simulink library "lib_GRM_HIL"  (R2019b)
settings: Solver=VariableStepAuto  StartTime=0.0  StopTime=10.0  RelTol=1e-3
values from neighbouring files (symbols this model uses):
  HIL_Sample_Time = 0.001    [initialize_GRM_HIL.m]
undefined symbols (not defined in the file or in its folder): HIL_Data
libraries: simulink x4, lib_Servo x3, lib_Flight_Controller x3, lib_Gimbal x3, lib_Encoder x2, lib_Serial_PIX x2, lib_Gimbal_Ctrl x2, lib_FDM x2, lib_Fin_Deflections x1, lib_Gimbal_Cmd x1, lib_IMU_GPS_Emulator x1, sldrtlib x1
settings Model: Creator=m.hiepp  LastModifiedBy=guy-m
settings DataIOCC: ReturnWorkspaceOutputs=off
settings DebuggingCC: ArithmeticOperatorsInVariantConditions=warning
settings SFSimCC: CustomCodeUndefinedFunction=UseInterfaceOnly

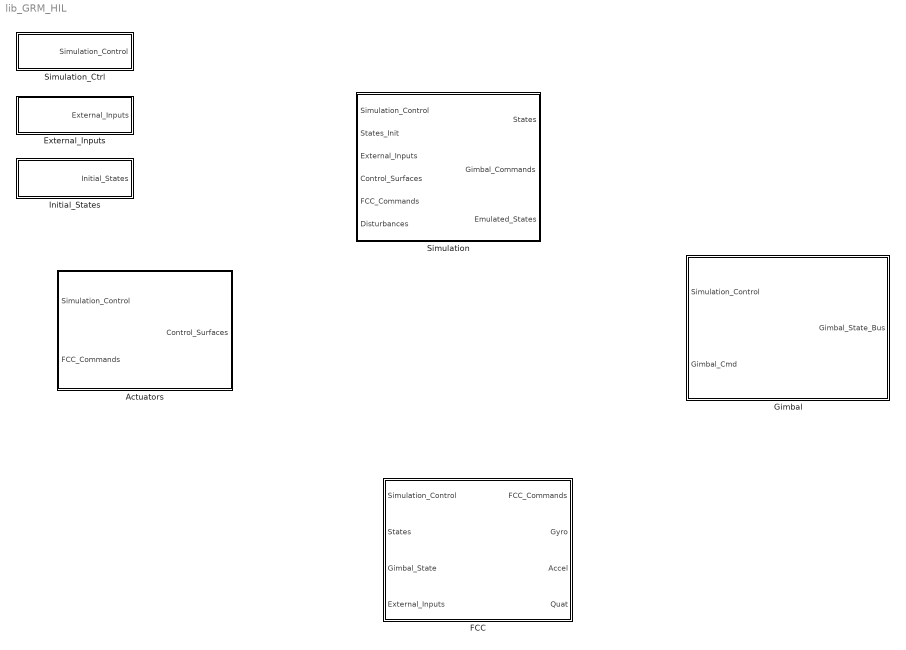
== system lib_GRM_HIL ==
  Actuators : Subsystem  Variant=on
  External_Inputs : Subsystem  mask{External_Inputs=HIL_Data.External_Inputs}
      mask prompts: External_Inputs "External Inputs Data"
  FCC : Subsystem  Variant=on
  Gimbal : Subsystem  Variant=on
  Initial_States : Subsystem  mask{Rigid_Body=HIL_Data.Initial_States.Rigid_Body, Airframe=HIL_Data.Initial_States.Airframe, Atm=HIL_Data.Initial_States.Atm}
      mask prompts: Rigid_Body "Rigid_Body Initial States Data"; Airframe "Airframe Initial States Data"; Atm "Atm Initial States Data"
  Simulation : Subsystem
  Simulation_Ctrl : Subsystem

== system lib_GRM_HIL/Actuators ==
  Simulation_Control : Inport  OutDataTypeStr=Bus: Simulation_Ctrl_Bus
  FCC_Commands : Inport  Port=2  OutDataTypeStr=Bus: FCC_Commands_Bus
  Emulate_Actuators : Subsystem  VariantControl=VSS_ACT_EMUL
  Use_Actuators : Subsystem  VariantControl=VSS_ACT_REAL
  Control_Surfaces : Outport  OutDataTypeStr=Bus: Control_Surface_Bus  VectorParamsAs1DForOutWhenUnconnected=off

== system lib_GRM_HIL/External_Inputs ==
  note: actually commanding roll rate instead of bank angle!!
  Bus Creator : BusCreator  Inputs=2  OutDataTypeStr=Bus: External_Inputs_Bus
  Bus Creator1 : BusCreator  Inputs=1  OutDataTypeStr=Bus: FDM_External_Inputs_Bus
  Bus Creator2 : BusCreator  Inputs=4  OutDataTypeStr=Bus: FCC_External_Inputs_Bus
  Commands_Generator : Subsystem
  Constant1 : Constant  Value=External_Inputs.FCC.Flight_Termination_flg  OutDataTypeStr=boolean
  Data Type Conversion : DataTypeConversion  OutDataTypeStr=boolean
  Step : Step  Time=External_Inputs.FDM.Motor_Ignition_time_s  SampleTime=0
  External_Inputs : Outport  OutDataTypeStr=Bus: External_Inputs_Bus  VectorParamsAs1DForOutWhenUnconnected=off
  wires:
  Bus Creator/1 -> External_Inputs/1
  Bus Creator1/1 -> Bus Creator/1  "FDM_External_Inputs_Bus"
  Bus Creator2/1 -> Bus Creator/2  "FCC_External_Inputs_Bus"
  Constant1/1 -> Bus Creator2/1  "Flight_Termination_flg"
  Step/1 -> Data Type Conversion/1
  Data Type Conversion/1 -> Bus Creator1/1  "Motor_Ignition_flg"
  Commands_Generator/3(CMD_acc_y_mDs2) -> Bus Creator2/4  "CMD_acc_y_mDs2"
  Commands_Generator/2(CMD_acc_z_mDs2) -> Bus Creator2/3  "CMD_acc_z_mDs2"
  Commands_Generator/1(CMD_phi_rad) -> Bus Creator2/2  "CMD_phi_rad"

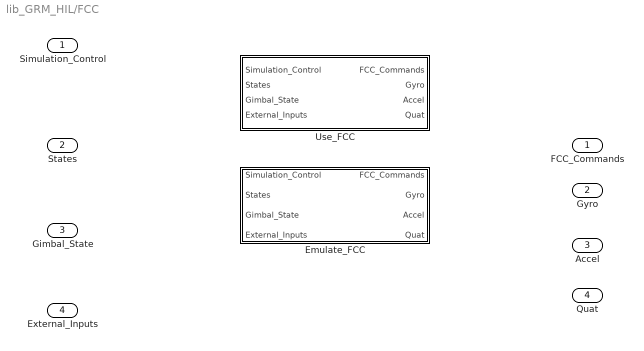
== system lib_GRM_HIL/FCC ==
  Simulation_Control : Inport  OutDataTypeStr=Bus: Simulation_Ctrl_Bus
  States : Inport  Port=2  OutDataTypeStr=Bus: States_Bus
  Gimbal_State : Inport  Port=3  OutDataTypeStr=Bus: Gimbal_State_Bus
  External_Inputs : Inport  Port=4  OutDataTypeStr=Bus: External_Inputs_Bus
  Emulate_FCC : Subsystem  VariantControl=VSS_FCC_EMUL
  Use_FCC : Subsystem  VariantControl=VSS_FCC_REAL
  FCC_Commands : Outport  OutDataTypeStr=Bus: FCC_Commands_Bus  VectorParamsAs1DForOutWhenUnconnected=off
  Gyro : Outport  Port=2
  Accel : Outport  Port=3
  Quat : Outport  Port=4

== system lib_GRM_HIL/Gimbal ==
  Simulation_Control : Inport  OutDataTypeStr=Bus: Simulation_Ctrl_Bus
  Gimbal_Cmd : Inport  Port=2  OutDataTypeStr=Bus: Gimbal_Cmd_Bus
  Emulate_Gimbal : Subsystem  VariantControl=VSS_GIMBAL_EMUL
  Use_Gimbal : Subsystem  VariantControl=VSS_GIMBAL_REAL
  Use_Gimbal_HWInterface_CC : Subsystem  VariantControl=VSS_GIMBAL_HWICC
  Gimbal_State_Bus : Outport  OutDataTypeStr=Bus: Gimbal_State_Bus  VectorParamsAs1DForOutWhenUnconnected=off

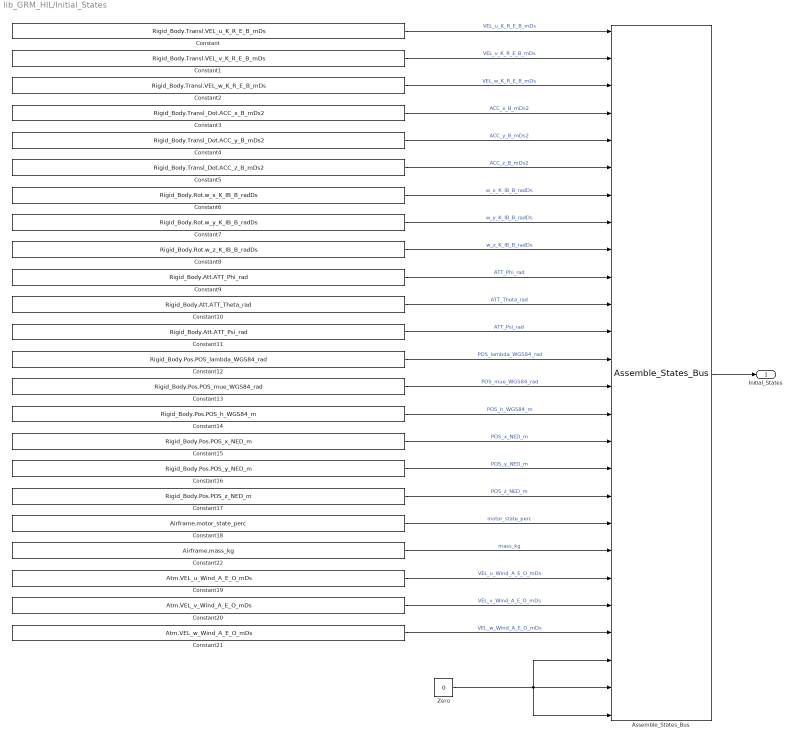
== system lib_GRM_HIL/Initial_States ==
  Assemble_States_Bus : lib_FDM/Assemble_States_Bus  SystemSampleTime=-1  Latency=0  AutoFrameSizeCalculation=off
  Constant : Constant  Value=Rigid_Body.Transl.VEL_u_K_R_E_B_mDs
  Constant1 : Constant  Value=Rigid_Body.Transl.VEL_v_K_R_E_B_mDs
  Constant10 : Constant  Value=Rigid_Body.Att.ATT_Theta_rad
  Constant11 : Constant  Value=Rigid_Body.Att.ATT_Psi_rad
  Constant12 : Constant  Value=Rigid_Body.Pos.POS_lambda_WGS84_rad
  Constant13 : Constant  Value=Rigid_Body.Pos.POS_mue_WGS84_rad
  Constant14 : Constant  Value=Rigid_Body.Pos.POS_h_WGS84_m
  Constant15 : Constant  Value=Rigid_Body.Pos.POS_x_NED_m
  Constant16 : Constant  Value=Rigid_Body.Pos.POS_y_NED_m
  Constant17 : Constant  Value=Rigid_Body.Pos.POS_z_NED_m
  Constant18 : Constant  Value=Airframe.motor_state_perc
  Constant19 : Constant  Value=Atm.VEL_u_Wind_A_E_O_mDs
  Constant2 : Constant  Value=Rigid_Body.Transl.VEL_w_K_R_E_B_mDs
  Constant20 : Constant  Value=Atm.VEL_v_Wind_A_E_O_mDs
  Constant21 : Constant  Value=Atm.VEL_w_Wind_A_E_O_mDs
  Constant22 : Constant  Value=Airframe.mass_kg
  Constant3 : Constant  Value=Rigid_Body.Transl_Dot.ACC_x_B_mDs2
  Constant4 : Constant  Value=Rigid_Body.Transl_Dot.ACC_y_B_mDs2
  Constant5 : Constant  Value=Rigid_Body.Transl_Dot.ACC_z_B_mDs2
  Constant6 : Constant  Value=Rigid_Body.Rot.w_x_K_IB_B_radDs
  Constant7 : Constant  Value=Rigid_Body.Rot.w_y_K_IB_B_radDs
  Constant8 : Constant  Value=Rigid_Body.Rot.w_z_K_IB_B_radDs
  Constant9 : Constant  Value=Rigid_Body.Att.ATT_Phi_rad
  Zero : Constant  Value=0  OutDataTypeStr=Inherit: Inherit via back propagation
  Initial_States : Outport  OutDataTypeStr=Bus: States_Bus  VectorParamsAs1DForOutWhenUnconnected=off
  wires:
  Assemble_States_Bus/1 -> Initial_States/1
  Constant/1 -> Assemble_States_Bus/1  "VEL_u_K_R_E_B_mDs"
  Constant1/1 -> Assemble_States_Bus/2  "VEL_v_K_R_E_B_mDs"
  Constant2/1 -> Assemble_States_Bus/3  "VEL_w_K_R_E_B_mDs"
  Constant4/1 -> Assemble_States_Bus/5  "ACC_y_B_mDs2"
  Constant3/1 -> Assemble_States_Bus/4  "ACC_x_B_mDs2"
  Constant5/1 -> Assemble_States_Bus/6  "ACC_z_B_mDs2"
  Constant6/1 -> Assemble_States_Bus/7  "w_x_K_IB_B_radDs"
  Constant7/1 -> Assemble_States_Bus/8  "w_y_K_IB_B_radDs"
  Constant8/1 -> Assemble_States_Bus/9  "w_z_K_IB_B_radDs"
  Constant9/1 -> Assemble_States_Bus/10  "ATT_Phi_rad"
  Constant10/1 -> Assemble_States_Bus/11  "ATT_Theta_rad"
  Constant11/1 -> Assemble_States_Bus/12  "ATT_Psi_rad"
  Constant12/1 -> Assemble_States_Bus/13  "POS_lambda_WGS84_rad"
  Constant13/1 -> Assemble_States_Bus/14  "POS_mue_WGS84_rad"
  Constant14/1 -> Assemble_States_Bus/15  "POS_h_WGS84_m"
  Constant15/1 -> Assemble_States_Bus/16  "POS_x_NED_m"
  Constant16/1 -> Assemble_States_Bus/17  "POS_y_NED_m"
  Constant17/1 -> Assemble_States_Bus/18  "POS_z_NED_m"
  Constant18/1 -> Assemble_States_Bus/19  "motor_state_perc"
  Constant19/1 -> Assemble_States_Bus/21  "VEL_u_Wind_A_E_O_mDs"
  Constant21/1 -> Assemble_States_Bus/23  "VEL_w_Wind_A_E_O_mDs"
  Constant20/1 -> Assemble_States_Bus/22  "VEL_v_Wind_A_E_O_mDs"
  Constant22/1 -> Assemble_States_Bus/20  "mass_kg"
  Zero/1 -> Assemble_States_Bus/26, Assemble_States_Bus/25, Assemble_States_Bus/24

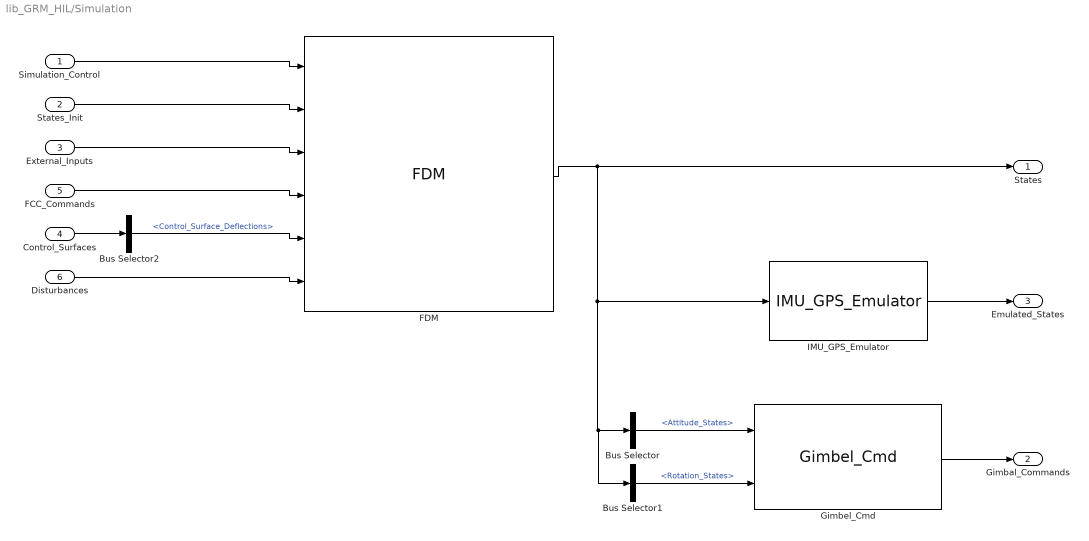
== system lib_GRM_HIL/Simulation ==
  Simulation_Control : Inport  OutDataTypeStr=Bus: Simulation_Ctrl_Bus
  States_Init : Inport  Port=2  OutDataTypeStr=Bus: States_Bus
  External_Inputs : Inport  Port=3  OutDataTypeStr=Bus: External_Inputs_Bus
  Control_Surfaces : Inport  Port=4  OutDataTypeStr=Bus: Control_Surface_Bus
  FCC_Commands : Inport  Port=5  OutDataTypeStr=Bus: FCC_Commands_Bus
  Disturbances : Inport  Port=6  OutDataTypeStr=Bus: Disturbances_Bus
  Bus Selector : BusSelector  OutputSignals=Rigid_Body_States.Attitude_States
  Bus Selector1 : BusSelector  OutputSignals=Rigid_Body_States.Rotation_States
  Bus Selector2 : BusSelector  OutputSignals=Control_Surface_Deflections
  FDM : lib_FDM/FDM  SystemSampleTime=-1  Latency=0  AutoFrameSizeCalculation=off
  Gimbel_Cmd : lib_Gimbal_Cmd/Gimbel_Cmd  SystemSampleTime=-1  Latency=0  AutoFrameSizeCalculation=off
  IMU_GPS_Emulator : lib_IMU_GPS_Emulator/IMU_GPS_Emulator  SystemSampleTime=-1  Latency=0  AutoFrameSizeCalculation=off
  States : Outport  OutDataTypeStr=Bus: States_Bus  VectorParamsAs1DForOutWhenUnconnected=off
  Gimbal_Commands : Outport  Port=2  OutDataTypeStr=Bus: Gimbal_Cmd_Bus  VectorParamsAs1DForOutWhenUnconnected=off
  Emulated_States : Outport  Port=3  OutDataTypeStr=Bus: States_Bus  VectorParamsAs1DForOutWhenUnconnected=off
  wires:
  FDM/1 -> Bus Selector/1, Bus Selector1/1, IMU_GPS_Emulator/1, States/1
  IMU_GPS_Emulator/1 -> Emulated_States/1
  Gimbel_Cmd/1 -> Gimbal_Commands/1
  Bus Selector/1 -> Gimbel_Cmd/1  "<Attitude_States>"
  Bus Selector1/1 -> Gimbel_Cmd/2  "<Rotation_States>"
  Simulation_Control/1 -> FDM/1
  States_Init/1 -> FDM/2
  External_Inputs/1 -> FDM/3
  FCC_Commands/1 -> FDM/4
  Control_Surfaces/1 -> Bus Selector2/1
  Bus Selector2/1 -> FDM/5  "<Control_Surface_Deflections>"
  Disturbances/1 -> FDM/6

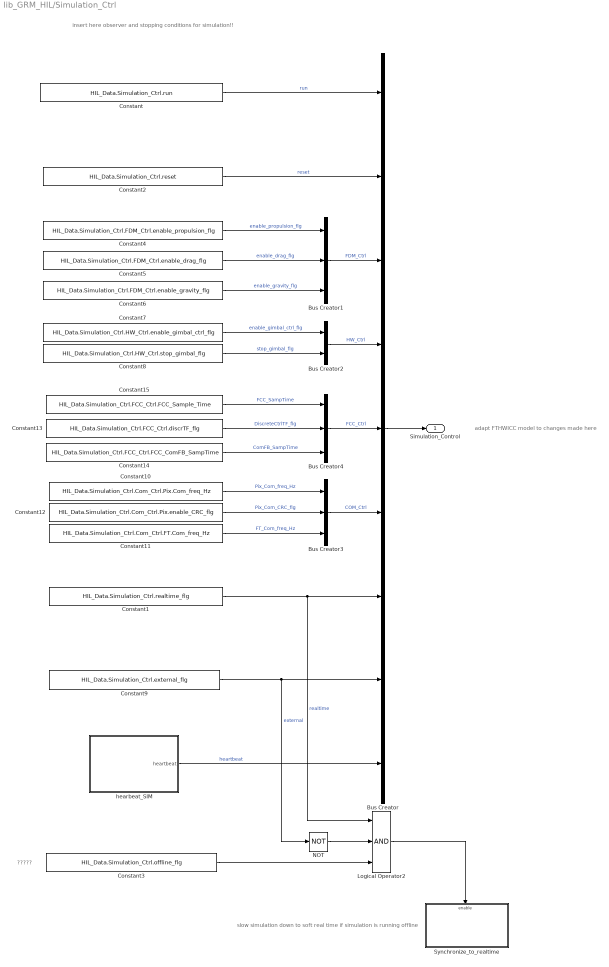
== system lib_GRM_HIL/Simulation_Ctrl ==
  note: adapt FTHWICC model to changes made here
  note: ?????
  note: slow simulation down to soft real time if simulation is running offline
  note: insert here observer and stopping conditions for simulation!!
  Bus Creator : BusCreator  Inputs=9  OutDataTypeStr=Bus: Simulation_Ctrl_Bus
  Bus Creator1 : BusCreator  Inputs=3  OutDataTypeStr=Bus: FDM_Ctrl_Bus
  Bus Creator2 : BusCreator  Inputs=2  OutDataTypeStr=Bus: HW_Ctrl_Bus
  Bus Creator3 : BusCreator  Inputs=3  OutDataTypeStr=Bus: COM_Ctrl_Bus
  Bus Creator4 : BusCreator  Inputs=3  OutDataTypeStr=Bus: FCC_Ctrl_Bus
  Constant : Constant  Value=HIL_Data.Simulation_Ctrl.run  OutDataTypeStr=boolean
  Constant1 : Constant  Value=HIL_Data.Simulation_Ctrl.realtime_flg  OutDataTypeStr=boolean
  Constant10 : Constant  Value=HIL_Data.Simulation_Ctrl.Com_Ctrl.Pix.Com_freq_Hz  OutDataTypeStr=double
  Constant11 : Constant  Value=HIL_Data.Simulation_Ctrl.Com_Ctrl.FT.Com_freq_Hz  OutDataTypeStr=double
  Constant12 : Constant  Value=HIL_Data.Simulation_Ctrl.Com_Ctrl.Pix.enable_CRC_flg  OutDataTypeStr=boolean
  Constant13 : Constant  Value=HIL_Data.Simulation_Ctrl.FCC_Ctrl.discrTF_flg  OutDataTypeStr=boolean
  Constant14 : Constant  Value=HIL_Data.Simulation_Ctrl.FCC_Ctrl.FCC_ComFB_SampTime  OutDataTypeStr=double
  Constant15 : Constant  Value=HIL_Data.Simulation_Ctrl.FCC_Ctrl.FCC_Sample_Time  OutDataTypeStr=double
  Constant2 : Constant  Value=HIL_Data.Simulation_Ctrl.reset  OutDataTypeStr=boolean
  Constant3 : Constant  Value=HIL_Data.Simulation_Ctrl.offline_flg  OutDataTypeStr=boolean
  Constant4 : Constant  Value=HIL_Data.Simulation_Ctrl.FDM_Ctrl.enable_propulsion_flg  OutDataTypeStr=boolean
  Constant5 : Constant  Value=HIL_Data.Simulation_Ctrl.FDM_Ctrl.enable_drag_flg  OutDataTypeStr=boolean
  Constant6 : Constant  Value=HIL_Data.Simulation_Ctrl.FDM_Ctrl.enable_gravity_flg  OutDataTypeStr=boolean
  Constant7 : Constant  Value=HIL_Data.Simulation_Ctrl.HW_Ctrl.enable_gimbal_ctrl_flg  OutDataTypeStr=double
  Constant8 : Constant  Value=HIL_Data.Simulation_Ctrl.HW_Ctrl.stop_gimbal_flg  OutDataTypeStr=double
  Constant9 : Constant  Value=HIL_Data.Simulation_Ctrl.external_flg  OutDataTypeStr=boolean
  Logical Operator2 : Logic  Inputs=3  AllPortsSameDT=off  OutDataTypeStr=boolean
  NOT : Logic  Operator=NOT  IconShape=distinctive  AllPortsSameDT=off  OutDataTypeStr=boolean
  Synchronize_to_realtime : Subsystem
  hearbeat_SIM : Subsystem  mask{heartbeat=HIL_Data.Simulation_Ctrl.heartbeat}
      mask prompts: heartbeat "Simulation heartbeat data"
  Simulation_Control : Outport  OutDataTypeStr=Bus: Simulation_Ctrl_Bus  VectorParamsAs1DForOutWhenUnconnected=off
  wires:
  Bus Creator/1 -> Simulation_Control/1
  Constant/1 -> Bus Creator/1  "run"
  Constant1/1 -> Logical Operator2/1, Bus Creator/7  "realtime"
  Constant2/1 -> Bus Creator/2  "reset"
  Constant3/1 -> Logical Operator2/3
  Logical Operator2/1 -> Synchronize_to_realtime/Enable
  Bus Creator1/1 -> Bus Creator/3  "FDM_Ctrl"
  Constant4/1 -> Bus Creator1/1  "enable_propulsion_flg"
  Constant5/1 -> Bus Creator1/2  "enable_drag_flg"
  Constant6/1 -> Bus Creator1/3  "enable_gravity_flg"
  Bus Creator2/1 -> Bus Creator/4  "HW_Ctrl"
  Constant8/1 -> Bus Creator2/2  "stop_gimbal_flg"
  Constant7/1 -> Bus Creator2/1  "enable_gimbal_ctrl_flg"
  Constant9/1 -> NOT/1, Bus Creator/8  "external"
  NOT/1 -> Logical Operator2/2
  Bus Creator3/1 -> Bus Creator/6  "COM_Ctrl"
  Constant11/1 -> Bus Creator3/3  "FT_Com_freq_Hz"
  Constant10/1 -> Bus Creator3/1  "Pix_Com_freq_Hz"
  hearbeat_SIM/1(heartbeat) -> Bus Creator/9  "heartbeat"
  Constant12/1 -> Bus Creator3/2  "Pix_Com_CRC_flg"
  Bus Creator4/1 -> Bus Creator/5  "FCC_Ctrl"
  Constant15/1 -> Bus Creator4/1  "FCC_SampTime"
  Constant13/1 -> Bus Creator4/2  "DiscreteCtrlTF_flg"
  Constant14/1 -> Bus Creator4/3  "ComFB_SampTime"

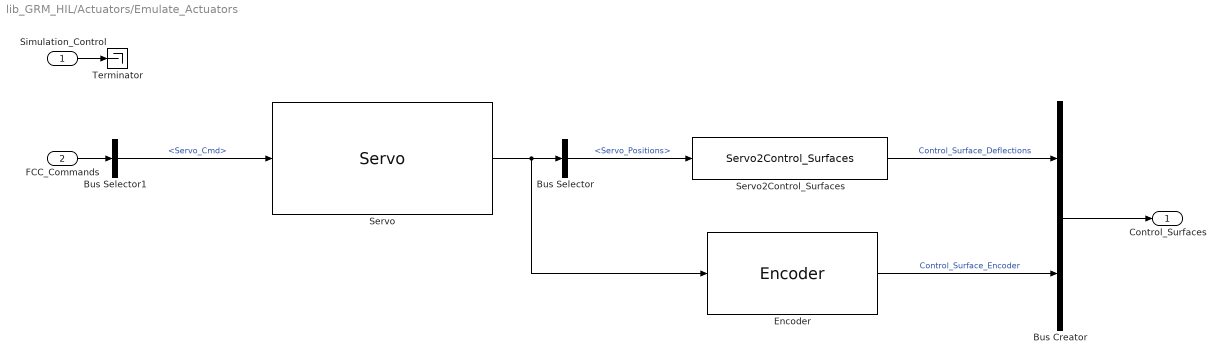
== system lib_GRM_HIL/Actuators/Emulate_Actuators ==
  Simulation_Control : Inport  OutDataTypeStr=Bus: Simulation_Ctrl_Bus
  FCC_Commands : Inport  Port=2  OutDataTypeStr=Bus: FCC_Commands_Bus
  Bus Creator : BusCreator  Inputs=2  OutDataTypeStr=Bus: Control_Surface_Bus
  Bus Selector : BusSelector  OutputSignals=Servo_Positions
  Bus Selector1 : BusSelector  OutputSignals=Airframe_Cmd.Servo_Cmd
  Encoder : lib_Encoder/Encoder  SystemSampleTime=-1  Latency=0  AutoFrameSizeCalculation=off
  Servo : lib_Servo/Servo  TF=HIL_Data.Servo.TF  PWM=HIL_Data.Servo.PWM
  Servo2Control_Surfaces : lib_Servo/Servo2Control_Surfaces  SystemSampleTime=-1  Latency=0  AutoFrameSizeCalculation=off
  Terminator : Terminator
  Control_Surfaces : Outport  OutDataTypeStr=Bus: Control_Surface_Bus  VectorParamsAs1DForOutWhenUnconnected=off
  wires:
  Encoder/1 -> Bus Creator/2  "Control_Surface_Encoder"
  Bus Creator/1 -> Control_Surfaces/1
  Bus Selector1/1 -> Servo/1  "<Servo_Cmd>"
  Servo2Control_Surfaces/1 -> Bus Creator/1  "Control_Surface_Deflections"
  Servo/1 -> Encoder/1, Bus Selector/1
  FCC_Commands/1 -> Bus Selector1/1
  Bus Selector/1 -> Servo2Control_Surfaces/1  "<Servo_Positions>"
  Simulation_Control/1 -> Terminator/1

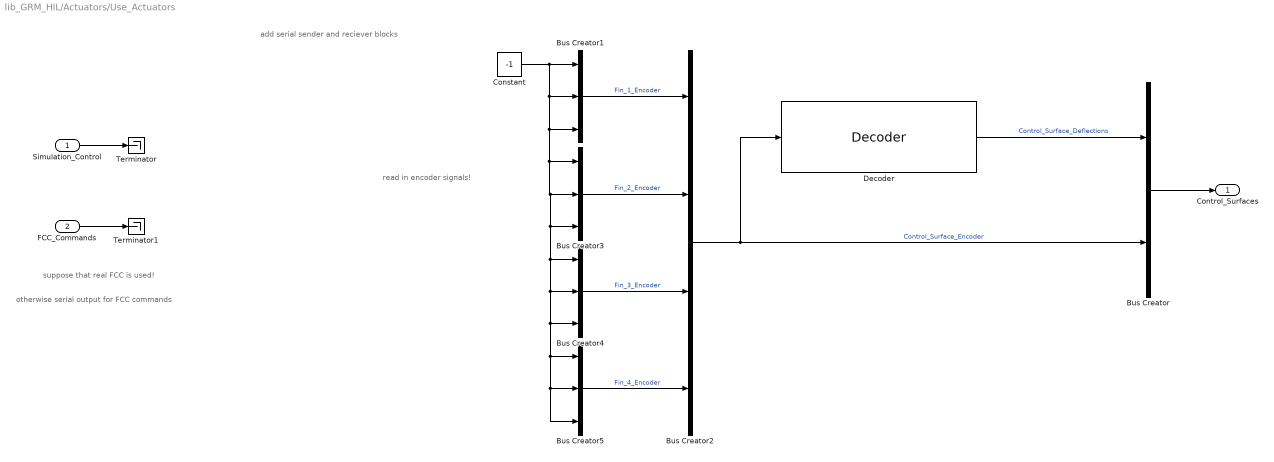
== system lib_GRM_HIL/Actuators/Use_Actuators ==
  note: read in encoder signals!
  note: otherwise serial output for FCC commands
  note: suppose that real FCC is used!
  note: add serial sender and reciever blocks
  Simulation_Control : Inport  OutDataTypeStr=Bus: Simulation_Ctrl_Bus
  FCC_Commands : Inport  Port=2  OutDataTypeStr=Bus: FCC_Commands_Bus
  Bus Creator : BusCreator  Inputs=2  OutDataTypeStr=Bus: Control_Surface_Bus
  Bus Creator{1,3..5} (4 alike) : BusCreator  Inputs=3  OutDataTypeStr=Bus: Inc_Encoder_Signal_Bus
  Bus Creator2 : BusCreator  Inputs=4  OutDataTypeStr=Bus: Control_Surface_Encoder_Bus
  Constant : Constant  Value=-1
  Decoder : lib_Encoder/Decoder  SystemSampleTime=-1  Latency=0  AutoFrameSizeCalculation=off
  Terminator : Terminator
  Terminator1 : Terminator
  Control_Surfaces : Outport  OutDataTypeStr=Bus: Control_Surface_Bus  VectorParamsAs1DForOutWhenUnconnected=off
  wires:
  Simulation_Control/1 -> Terminator/1
  FCC_Commands/1 -> Terminator1/1
  Bus Creator/1 -> Control_Surfaces/1
  Bus Creator2/1 -> Decoder/1, Bus Creator/2  "Control_Surface_Encoder"
  Bus Creator1/1 -> Bus Creator2/1  "Fin_1_Encoder"
  Bus Creator3/1 -> Bus Creator2/2  "Fin_2_Encoder"
  Bus Creator5/1 -> Bus Creator2/4  "Fin_4_Encoder"
  Bus Creator4/1 -> Bus Creator2/3  "Fin_3_Encoder"
  Decoder/1 -> Bus Creator/1  "Control_Surface_Deflections"
  Constant/1 -> Bus Creator4/1, Bus Creator5/1, Bus Creator5/3, Bus Creator5/2, Bus Creator4/3, Bus Creator4/2, Bus Creator3/3, Bus Creator3/2, Bus Creator3/1, Bus Creator1/3, Bus Creator1/2, Bus Creator1/1

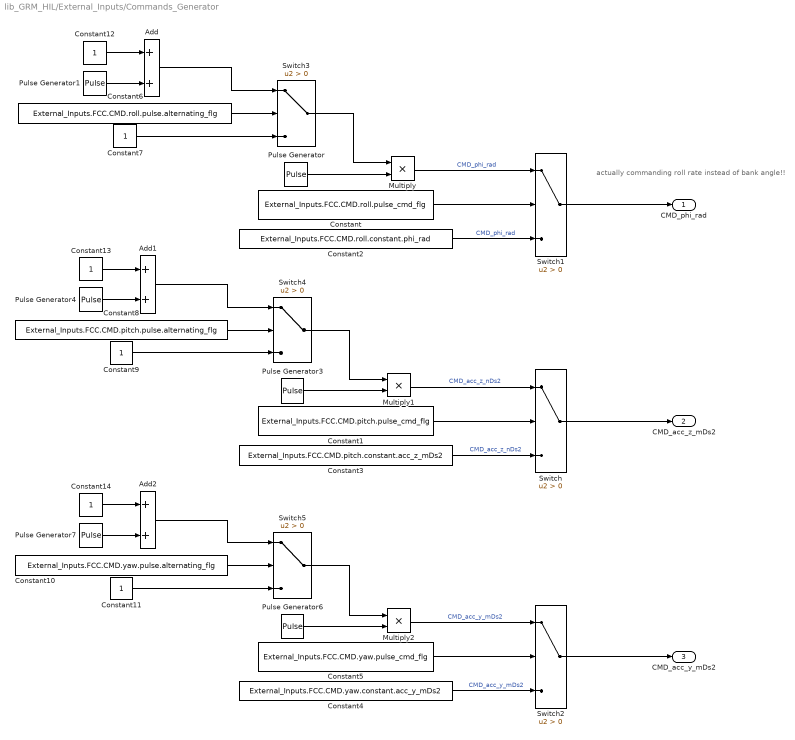
== system lib_GRM_HIL/External_Inputs/Commands_Generator ==
  note: actually commanding roll rate instead of bank angle!!
  Add : Sum
  Add1 : Sum
  Add2 : Sum
  Constant : Constant  Value=External_Inputs.FCC.CMD.roll.pulse_cmd_flg
  Constant1 : Constant  Value=External_Inputs.FCC.CMD.pitch.pulse_cmd_flg
  Constant10 : Constant  Value=External_Inputs.FCC.CMD.yaw.pulse.alternating_flg  OutDataTypeStr=boolean
  Constant{7,9,11..14} (6 alike) : Constant
  Constant2 : Constant  Value=External_Inputs.FCC.CMD.roll.constant.phi_rad
  Constant3 : Constant  Value=External_Inputs.FCC.CMD.pitch.constant.acc_z_mDs2
  Constant4 : Constant  Value=External_Inputs.FCC.CMD.yaw.constant.acc_y_mDs2
  Constant5 : Constant  Value=External_Inputs.FCC.CMD.yaw.pulse_cmd_flg
  Constant6 : Constant  Value=External_Inputs.FCC.CMD.roll.pulse.alternating_flg  OutDataTypeStr=boolean
  Constant8 : Constant  Value=External_Inputs.FCC.CMD.pitch.pulse.alternating_flg  OutDataTypeStr=boolean
  Multiply : Product
  Multiply1 : Product
  Multiply2 : Product
  Pulse Generator : DiscretePulseGenerator  PulseType=Time based  Amplitude=External_Inputs.FCC.CMD.roll.pulse.ampl_rad  Period=External_Inputs.FCC.CMD.roll.pulse.period_s  PulseWidth=External_Inputs.FCC.CMD.roll.pulse.pulse_width_perc  PhaseDelay=External_Inputs.FCC.CMD.roll.pulse.delay_s
  Pulse Generator1 : DiscretePulseGenerator  PulseType=Time based  Amplitude=-2  Period=2*External_Inputs.FCC.CMD.roll.pulse.period_s  PulseWidth=External_Inputs.FCC.CMD.roll.pulse.pulse_width_perc  PhaseDelay=External_Inputs.FCC.CMD.roll.pulse.delay_s+External_Inputs.FCC.CMD.roll.pulse.period_s
  Pulse Generator3 : DiscretePulseGenerator  PulseType=Time based  Amplitude=External_Inputs.FCC.CMD.pitch.pulse.ampl_mDs2  Period=External_Inputs.FCC.CMD.pitch.pulse.period_s  PulseWidth=External_Inputs.FCC.CMD.pitch.pulse.pulse_width_perc  PhaseDelay=External_Inputs.FCC.CMD.pitch.pulse.delay_s
  Pulse Generator4 : DiscretePulseGenerator  PulseType=Time based  Amplitude=-2  Period=2*External_Inputs.FCC.CMD.pitch.pulse.period_s  PulseWidth=External_Inputs.FCC.CMD.pitch.pulse.pulse_width_perc  PhaseDelay=External_Inputs.FCC.CMD.pitch.pulse.delay_s+External_Inputs.FCC.CMD.pitch.pulse.period_s
  Pulse Generator6 : DiscretePulseGenerator  PulseType=Time based  Amplitude=External_Inputs.FCC.CMD.yaw.pulse.ampl_mDs2  Period=External_Inputs.FCC.CMD.yaw.pulse.period_s  PulseWidth=External_Inputs.FCC.CMD.yaw.pulse.pulse_width_perc  PhaseDelay=External_Inputs.FCC.CMD.yaw.pulse.delay_s
  Pulse Generator7 : DiscretePulseGenerator  PulseType=Time based  Amplitude=-2  Period=2*External_Inputs.FCC.CMD.yaw.pulse.period_s  PulseWidth=External_Inputs.FCC.CMD.yaw.pulse.pulse_width_perc  PhaseDelay=External_Inputs.FCC.CMD.yaw.pulse.delay_s+External_Inputs.FCC.CMD.yaw.pulse.period_s
  Switch{,1..5} (6 alike) : Switch  Criteria=u2 > Threshold
  CMD_phi_rad : Outport  VectorParamsAs1DForOutWhenUnconnected=off
  CMD_acc_z_mDs2 : Outport  Port=2  VectorParamsAs1DForOutWhenUnconnected=off
  CMD_acc_y_mDs2 : Outport  Port=3  VectorParamsAs1DForOutWhenUnconnected=off
  wires:
  Switch/1 -> CMD_acc_z_mDs2/1
  Switch1/1 -> CMD_phi_rad/1
  Switch2/1 -> CMD_acc_y_mDs2/1
  Constant2/1 -> Switch1/3  "CMD_phi_rad"
  Constant4/1 -> Switch2/3  "CMD_acc_y_mDs2"
  Constant3/1 -> Switch/3  "CMD_acc_z_nDs2"
  Constant/1 -> Switch1/2
  Constant1/1 -> Switch/2
  Constant5/1 -> Switch2/2
  Constant6/1 -> Switch3/2
  Constant7/1 -> Switch3/3
  Constant12/1 -> Add/1
  Pulse Generator1/1 -> Add/2
  Add/1 -> Switch3/1
  Multiply/1 -> Switch1/1  "CMD_phi_rad"
  Pulse Generator/1 -> Multiply/2
  Switch3/1 -> Multiply/1
  Switch4/1 -> Multiply1/1
  Constant8/1 -> Switch4/2
  Pulse Generator3/1 -> Multiply1/2
  Pulse Generator4/1 -> Add1/2
  Constant9/1 -> Switch4/3
  Constant13/1 -> Add1/1
  Add1/1 -> Switch4/1
  Multiply1/1 -> Switch/1  "CMD_acc_z_nDs2"
  Switch5/1 -> Multiply2/1
  Constant10/1 -> Switch5/2
  Pulse Generator6/1 -> Multiply2/2
  Pulse Generator7/1 -> Add2/2
  Constant11/1 -> Switch5/3
  Constant14/1 -> Add2/1
  Add2/1 -> Switch5/1
  Multiply2/1 -> Switch2/1  "CMD_acc_y_mDs2"

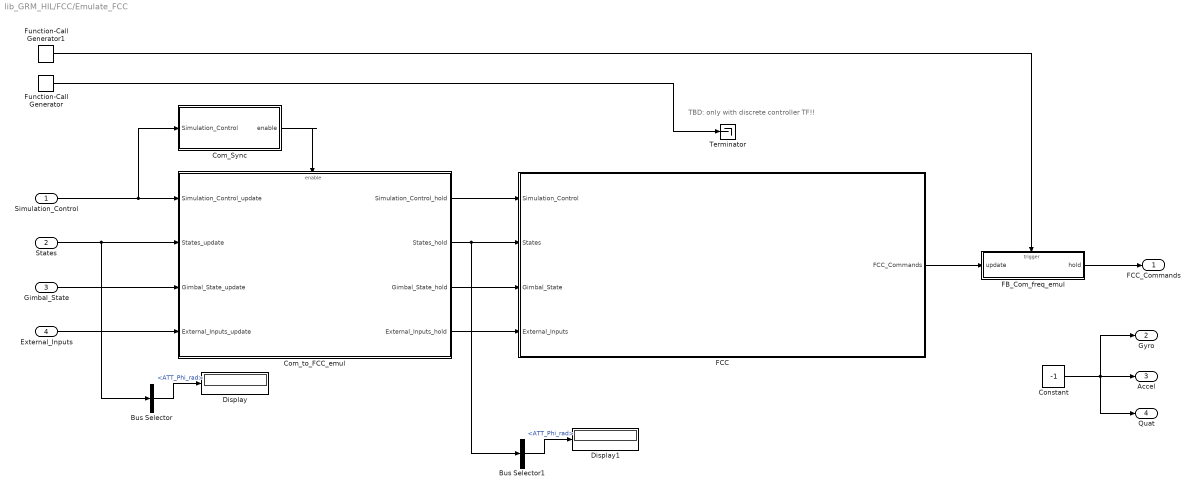
== system lib_GRM_HIL/FCC/Emulate_FCC ==
  note: TBD: only with discrete controller TF!!
  Simulation_Control : Inport  OutDataTypeStr=Bus: Simulation_Ctrl_Bus
  States : Inport  Port=2  OutDataTypeStr=Bus: States_Bus
  Gimbal_State : Inport  Port=3  OutDataTypeStr=Bus: Gimbal_State_Bus
  External_Inputs : Inport  Port=4  OutDataTypeStr=Bus: External_Inputs_Bus
  Bus Selector : BusSelector  OutputSignals=Rigid_Body_States.Attitude_States.ATT_Euler.ATT_Phi_rad
  Bus Selector1 : BusSelector  OutputSignals=Rigid_Body_States.Attitude_States.ATT_Euler.ATT_Phi_rad
  Com_Sync : Subsystem
  Com_to_FCC_emul : Subsystem
  Constant : Constant  Value=-1
  Display : Display
  Display1 : Display
  FB_Com_freq_emul : Subsystem
  FCC : Subsystem
  Function-Call Generator : simulink/Ports & Subsystems/Function-Call Generator  sample_time=HIL_Data.Simulation_Ctrl.FCC_Ctrl.FCC_Sample_Time  numberOfIterations=1
  Function-Call Generator1 : simulink/Ports & Subsystems/Function-Call Generator  sample_time=HIL_Data.Simulation_Ctrl.FCC_Ctrl.FCC_ComFB_SampTime  numberOfIterations=1
  Terminator : Terminator
  FCC_Commands : Outport  OutDataTypeStr=Bus: FCC_Commands_Bus  VectorParamsAs1DForOutWhenUnconnected=off
  Gyro : Outport  Port=2
  Accel : Outport  Port=3
  Quat : Outport  Port=4
  wires:
  Simulation_Control/1 -> Com_to_FCC_emul/1(Simulation_Control_update), Com_Sync/1(Simulation_Control)
  Function-Call Generator/1 -> Terminator/1
  FB_Com_freq_emul/1(hold) -> FCC_Commands/1
  FCC/1(FCC_Commands) -> FB_Com_freq_emul/1(update)
  Com_to_FCC_emul/4(External_Inputs_hold) -> FCC/4(External_Inputs)
  Com_to_FCC_emul/3(Gimbal_State_hold) -> FCC/3(Gimbal_State)
  Com_to_FCC_emul/1(Simulation_Control_hold) -> FCC/1(Simulation_Control)
  States/1 -> Bus Selector/1, Com_to_FCC_emul/2(States_update)
  Gimbal_State/1 -> Com_to_FCC_emul/3(Gimbal_State_update)
  External_Inputs/1 -> Com_to_FCC_emul/4(External_Inputs_update)
  Com_Sync/1(enable) -> Com_to_FCC_emul/Enable
  Function-Call Generator1/1 -> FB_Com_freq_emul/Trigger
  Bus Selector/1 -> Display/1  "<ATT_Phi_rad>"
  Bus Selector1/1 -> Display1/1  "<ATT_Phi_rad>"
  Com_to_FCC_emul/2(States_hold) -> Bus Selector1/1, FCC/2(States)
  Constant/1 -> Quat/1, Accel/1, Gyro/1

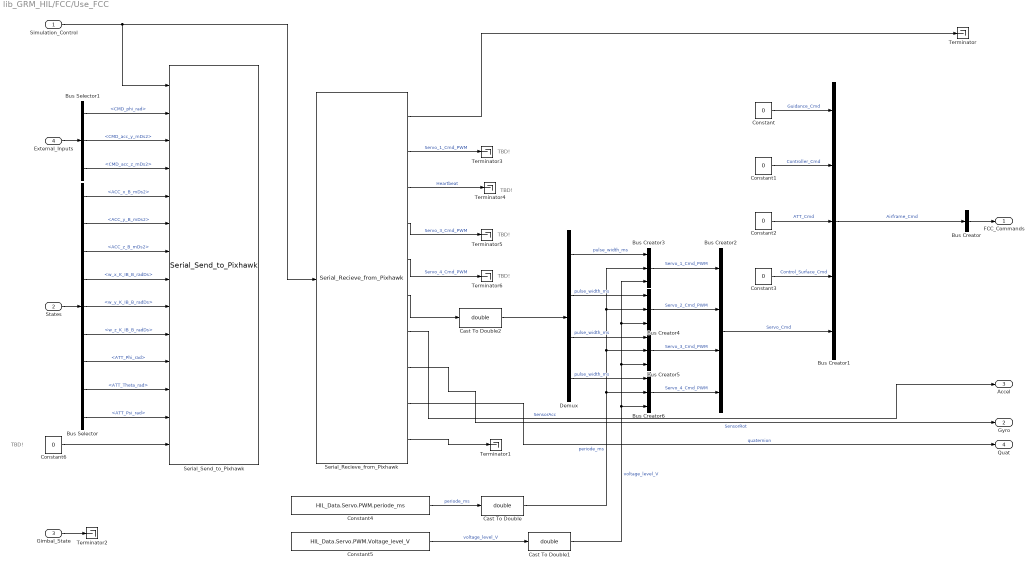
== system lib_GRM_HIL/FCC/Use_FCC ==
  note: TBD!
  note: TBD!
  note: TBD!
  note: TBD!
  note: TBD!
  Simulation_Control : Inport  OutDataTypeStr=Bus: Simulation_Ctrl_Bus
  States : Inport  Port=2  OutDataTypeStr=Bus: States_Bus
  Gimbal_State : Inport  Port=3  OutDataTypeStr=Bus: Gimbal_State_Bus
  External_Inputs : Inport  Port=4  OutDataTypeStr=Bus: External_Inputs_Bus
  Bus Creator : BusCreator  Inputs=1  OutDataTypeStr=Bus: FCC_Commands_Bus
  Bus Creator1 : BusCreator  Inputs=5  OutDataTypeStr=Bus: Airframe_Cmd_Bus
  Bus Creator2 : BusCreator  Inputs=4  OutDataTypeStr=Bus: Servo_Cmd_Bus
  Bus Creator{3..6} (4 alike) : BusCreator  Inputs=3  OutDataTypeStr=Bus: PWM_Cmd_Bus
  Bus Selector : BusSelector  OutputSignals=Rigid_Body_States.Acceleration_States.ACC_x_B_mDs2,Rigid_Body_States.Acceleration_States.ACC_y_B_mDs2,Rigid_Body_States.Acceleration_States.ACC_z_B_mDs2,Rigid_Body_States.Rotation_States.w_x_K_IB_B_radDs,Rigid_Body_States.Rotation_States.w_y_K_IB_B_radDs,Rigid_Body_States.Rotation_States.w_z_K_IB_B_radDs,Rigid_Body_States.Attitude_States.ATT_Euler.ATT_Phi_rad,Rigid_Body_States.Attitude_States.ATT_Euler.ATT_Theta_rad,Rigid_Body_States.Attitude_States.ATT_Euler.ATT_Psi_rad
  Bus Selector1 : BusSelector  OutputSignals=FCC_External_Inputs.CMD_phi_rad,FCC_External_Inputs.CMD_acc_y_mDs2,FCC_External_Inputs.CMD_acc_z_mDs2
  Cast To Double : DataTypeConversion  OutDataTypeStr=double
  Cast To Double1 : DataTypeConversion  OutDataTypeStr=double
  Cast To Double2 : DataTypeConversion  OutDataTypeStr=double
  Constant : Constant  Value=0  OutDataTypeStr=Bus: Guidance_Cmd_Bus
  Constant1 : Constant  Value=0  OutDataTypeStr=Bus: Controller_Cmd_Bus
  Constant2 : Constant  Value=0  OutDataTypeStr=Bus: ATT_Cmd_Bus
  Constant3 : Constant  Value=0  OutDataTypeStr=Bus: Control_Surface_Cmd_Bus
  Constant4 : Constant  Value=HIL_Data.Servo.PWM.periode_ms
  Constant5 : Constant  Value=HIL_Data.Servo.PWM.Voltage_level_V
  Constant6 : Constant  Value=0  OutDataTypeStr=single
  Demux : Demux
  Serial_Recieve_from_Pixhawk : lib_Serial_PIX/Serial_Recieve_from_Pixhawk  Serial=HIL_Data.Serial.Pix
  Serial_Send_to_Pixhawk : lib_Serial_PIX/Serial_Send_to_Pixhawk  Serial=HIL_Data.Serial.Pix
  Terminator{,1..6} (7 alike) : Terminator
  FCC_Commands : Outport  OutDataTypeStr=Bus: FCC_Commands_Bus  VectorParamsAs1DForOutWhenUnconnected=off
  Gyro : Outport  Port=2
  Accel : Outport  Port=3
  Quat : Outport  Port=4
  wires:
  Constant/1 -> Bus Creator1/1  "Guidance_Cmd"
  Constant1/1 -> Bus Creator1/2  "Controller_Cmd"
  Bus Creator1/1 -> Bus Creator/1  "Airframe_Cmd"
  Constant2/1 -> Bus Creator1/3  "ATT_Cmd"
  Bus Creator2/1 -> Bus Creator1/5  "Servo_Cmd"
  Bus Creator/1 -> FCC_Commands/1
  Constant3/1 -> Bus Creator1/4  "Control_Surface_Cmd"
  Serial_Recieve_from_Pixhawk/1 -> Terminator/1
  Gimbal_State/1 -> Terminator2/1
  External_Inputs/1 -> Bus Selector1/1
  States/1 -> Bus Selector/1
  Bus Creator3/1 -> Bus Creator2/1  "Servo_1_Cmd_PWM"
  Bus Creator4/1 -> Bus Creator2/2  "Servo_2_Cmd_PWM"
  Bus Creator5/1 -> Bus Creator2/3  "Servo_3_Cmd_PWM"
  Bus Creator6/1 -> Bus Creator2/4  "Servo_4_Cmd_PWM"
  Demux/1 -> Bus Creator3/1  "pulse_width_ms"
  Demux/2 -> Bus Creator4/1  "pulse_width_ms"
  Demux/3 -> Bus Creator5/1  "pulse_width_ms"
  Demux/4 -> Bus Creator6/1  "pulse_width_ms"
  Constant4/1 -> Cast To Double/1  "periode_ms"
  Constant5/1 -> Cast To Double1/1  "voltage_level_V"
  Serial_Recieve_from_Pixhawk/6 -> Cast To Double2/1
  Serial_Recieve_from_Pixhawk/2 -> Terminator3/1  "Servo_1_Cmd_PWM"
  Serial_Recieve_from_Pixhawk/3 -> Terminator4/1  "Heartbeat"
  Serial_Recieve_from_Pixhawk/4 -> Terminator5/1  "Servo_3_Cmd_PWM"
  Serial_Recieve_from_Pixhawk/5 -> Terminator6/1  "Servo_4_Cmd_PWM"
  Serial_Recieve_from_Pixhawk/7 -> Accel/1  "SensorAcc"
  Serial_Recieve_from_Pixhawk/8 -> Gyro/1  "SensorRot"
  Serial_Recieve_from_Pixhawk/9 -> Quat/1  "quaternion"
  Bus Selector1/1 -> Serial_Send_to_Pixhawk/2  "<CMD_phi_rad>"
  Bus Selector1/2 -> Serial_Send_to_Pixhawk/3  "<CMD_acc_y_mDs2>"
  Bus Selector1/3 -> Serial_Send_to_Pixhawk/4  "<CMD_acc_z_mDs2>"
  Bus Selector/1 -> Serial_Send_to_Pixhawk/5  "<ACC_x_B_mDs2>"
  Bus Selector/2 -> Serial_Send_to_Pixhawk/6  "<ACC_y_B_mDs2>"
  Bus Selector/3 -> Serial_Send_to_Pixhawk/7  "<ACC_z_B_mDs2>"
  Bus Selector/4 -> Serial_Send_to_Pixhawk/8  "<w_x_K_IB_B_radDs>"
  Bus Selector/5 -> Serial_Send_to_Pixhawk/9  "<w_y_K_IB_B_radDs>"
  Bus Selector/6 -> Serial_Send_to_Pixhawk/10  "<w_z_K_IB_B_radDs>"
  Bus Selector/7 -> Serial_Send_to_Pixhawk/11  "<ATT_Phi_rad>"
  Bus Selector/8 -> Serial_Send_to_Pixhawk/12  "<ATT_Theta_rad>"
  Bus Selector/9 -> Serial_Send_to_Pixhawk/13  "<ATT_Psi_rad>"
  Simulation_Control/1 -> Serial_Send_to_Pixhawk/1, Serial_Recieve_from_Pixhawk/1
  Constant6/1 -> Serial_Send_to_Pixhawk/14
  Cast To Double/1 -> Bus Creator6/2, Bus Creator5/2, Bus Creator4/2, Bus Creator3/2  "periode_ms"
  Cast To Double1/1 -> Bus Creator6/3, Bus Creator5/3, Bus Creator4/3, Bus Creator3/3  "voltage_level_V"
  Cast To Double2/1 -> Demux/1
  Serial_Recieve_from_Pixhawk/10 -> Terminator1/1

== system lib_GRM_HIL/Gimbal/Emulate_Gimbal ==
  Simulation_Control : Inport  OutDataTypeStr=Bus: Simulation_Ctrl_Bus
  Gimbal_Cmd : Inport  Port=2  OutDataTypeStr=Bus: Gimbal_Cmd_Bus
  Bus Creator : BusCreator  Inputs=3  OutDataTypeStr=Bus: Gimbal_State_Bus
  Gimbal : lib_Gimbal/Gimbal  SystemSampleTime=-1  Latency=0  AutoFrameSizeCalculation=off
  Gimbel_Ctrl : lib_Gimbal_Ctrl/Gimbel_Ctrl  Gimbal_Ctrl=HIL_Data.Gimbal_Ctrl  SampTime=HIL_Data.Gimbal_Ctrl.SampTime
  Memory : Memory  InheritSampleTime=on  LinearizeAsDelay=on
  Memory1 : Memory  InheritSampleTime=on  LinearizeAsDelay=on
  Gimbal_State_Bus : Outport  OutDataTypeStr=Bus: Gimbal_State_Bus  VectorParamsAs1DForOutWhenUnconnected=off
  wires:
  Bus Creator/1 -> Gimbal_State_Bus/1
  Gimbal/2 -> Memory1/1, Bus Creator/3  "Gimbal_Encoder_Bus"
  Gimbal/1 -> Bus Creator/2  "Gimbal_Attitude_Bus"
  Gimbel_Ctrl/2 -> Gimbal/1
  Gimbel_Ctrl/1 -> Bus Creator/1  "Gimbal_Status_Bus"
  Simulation_Control/1 -> Gimbel_Ctrl/1
  Gimbal_Cmd/1 -> Gimbel_Ctrl/2
  Gimbal/3 -> Memory/1
  Memory/1 -> Gimbel_Ctrl/4
  Memory1/1 -> Gimbel_Ctrl/3

== system lib_GRM_HIL/Gimbal/Use_Gimbal ==
  Simulation_Control : Inport  OutDataTypeStr=Bus: Simulation_Ctrl_Bus
  Gimbal_Cmd : Inport  Port=2  OutDataTypeStr=Bus: Gimbal_Cmd_Bus
  Bus Creator : BusCreator  Inputs=3  OutDataTypeStr=Bus: Gimbal_State_Bus
  Gimbal_HW_Interface : lib_Gimbal/Gimbal_HW_Interface  HW=HIL_Data.Gimbal.HW
  Gimbel_Ctrl : lib_Gimbal_Ctrl/Gimbel_Ctrl  Gimbal_Ctrl=HIL_Data.Gimbal_Ctrl  SampTime=HIL_Data.Gimbal_Ctrl.SampTime
  Gimbal_State_Bus : Outport  OutDataTypeStr=Bus: Gimbal_State_Bus  VectorParamsAs1DForOutWhenUnconnected=off
  wires:
  Bus Creator/1 -> Gimbal_State_Bus/1
  Gimbal_HW_Interface/1 -> Bus Creator/2  "Gimbal_Attitude_Bus"
  Gimbel_Ctrl/1 -> Bus Creator/1  "Gimbal_Status_Bus"
  Gimbal_HW_Interface/2 -> Gimbel_Ctrl/3, Bus Creator/3  "Gimbal_Encoder_Bus"
  Simulation_Control/1 -> Gimbel_Ctrl/1
  Gimbal_Cmd/1 -> Gimbel_Ctrl/2
  Gimbel_Ctrl/2 -> Gimbal_HW_Interface/1
  Gimbal_HW_Interface/3 -> Gimbel_Ctrl/4

== system lib_GRM_HIL/Gimbal/Use_Gimbal_HWInterface_CC ==
  Simulation_Control : Inport  OutDataTypeStr=Bus: Simulation_Ctrl_Bus
  Gimbal_Cmd : Inport  Port=2  OutDataTypeStr=Bus: Gimbal_Cmd_Bus
  Bus Creator : BusCreator  Inputs=3  OutDataTypeStr=Bus: Gimbal_State_Bus
  Communication_FT_HWI_ControlComputer : lib_Gimbal/Communication_FT_HWI_ControlComputer  HW=HIL_Data.Gimbal.HW
  Gimbal_State_Bus : Outport  OutDataTypeStr=Bus: Gimbal_State_Bus  VectorParamsAs1DForOutWhenUnconnected=off
  wires:
  Bus Creator/1 -> Gimbal_State_Bus/1
  Communication_FT_HWI_ControlComputer/3 -> Bus Creator/3  "Gimbal_Encoder_Bus"
  Communication_FT_HWI_ControlComputer/2 -> Bus Creator/2  "Gimbal_Attitude_Bus"
  Communication_FT_HWI_ControlComputer/1 -> Bus Creator/1  "Gimbal_Status_Bus"
  Simulation_Control/1 -> Communication_FT_HWI_ControlComputer/1
  Gimbal_Cmd/1 -> Communication_FT_HWI_ControlComputer/2

== system lib_GRM_HIL/Simulation_Ctrl/Synchronize_to_realtime ==
  Enable : EnablePort
  Real-Time Synchronization : sldrtlib/Real-Time Synchronization  SampleTime=HIL_Sample_Time  MaxMissedTicks=1000  ShowMissedTicks=off  YieldWhenWaiting=off

== system lib_GRM_HIL/Simulation_Ctrl/hearbeat_SIM ==
  Add7 : Sum  Commented=on
  Constant6 : Constant  Commented=on
  Counter Free-Running : simulink/Sources/Counter Free-Running  NumBits=heartbeat.range  tsamp=HIL_Sample_Time
  Counter Limited : simulink/Sources/Counter Limited  Commented=on  uplimit=50000  tsamp=-1
  Data Type Conversion1 : DataTypeConversion  OutDataTypeStr=uint16
  Data Type Conversion6 : DataTypeConversion  Commented=on  OutDataTypeStr=uint16
  IC : InitialCondition  Commented=on  Value=0
  Memory : Memory  Commented=on  InheritSampleTime=on
  heartbeat : Outport  VectorParamsAs1DForOutWhenUnconnected=off
  wires:
  Add7/1 -> Memory/1
  IC/1 -> Add7/2
  Memory/1 -> IC/1
  Constant6/1 -> Add7/1
  Counter Limited/1 -> Data Type Conversion6/1
  Counter Free-Running/1 -> Data Type Conversion1/1
  Data Type Conversion1/1 -> heartbeat/1

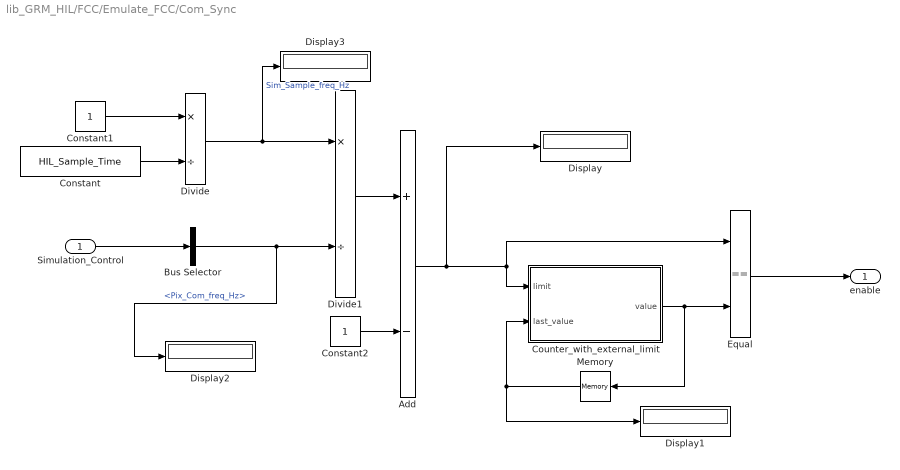
== system lib_GRM_HIL/FCC/Emulate_FCC/Com_Sync ==
  Simulation_Control : Inport  OutDataTypeStr=Bus: Simulation_Ctrl_Bus
  Add : Sum  Inputs=+-
  Bus Selector : BusSelector  OutputSignals=COM_Ctrl.Pix_Com_freq_Hz
  Constant : Constant  Value=HIL_Sample_Time
  Constant1 : Constant
  Constant2 : Constant
  Counter_with_external_limit : MATLAB Function  TreatAsAtomicUnit=on
  Display{,1..3} (4 alike) : Display
  Divide : Product  Inputs=*/
  Divide1 : Product  Inputs=*/
  Equal : RelationalOperator  Operator===  OutDataTypeStr=boolean  RndMeth=Simplest
  Memory : Memory  InitialCondition=-1
  enable : Outport  VectorParamsAs1DForOutWhenUnconnected=off
  wires:
  Equal/1 -> enable/1
  Simulation_Control/1 -> Bus Selector/1
  Constant/1 -> Divide/2
  Constant1/1 -> Divide/1
  Divide/1 -> Display3/1, Divide1/1  "Sim_Sample_freq_Hz"
  Bus Selector/1 -> Display2/1, Divide1/2  "<Pix_Com_freq_Hz>"
  Divide1/1 -> Add/1
  Constant2/1 -> Add/2
  Counter_with_external_limit/1(value) -> Memory/1, Equal/2
  Add/1 -> Display/1, Equal/1, Counter_with_external_limit/1(limit)
  Memory/1 -> Counter_with_external_limit/2(last_value), Display1/1

== system lib_GRM_HIL/FCC/Emulate_FCC/Com_to_FCC_emul ==
  Simulation_Control_update : Inport  OutDataTypeStr=Bus: Simulation_Ctrl_Bus
  States_update : Inport  Port=2  OutDataTypeStr=Bus: States_Bus
  Gimbal_State_update : Inport  Port=3  OutDataTypeStr=Bus: Gimbal_State_Bus
  External_Inputs_update : Inport  Port=4  OutDataTypeStr=Bus: External_Inputs_Bus
  Enable : EnablePort
  Simulation_Control_hold : Outport  OutDataTypeStr=Bus: Simulation_Ctrl_Bus  VectorParamsAs1DForOutWhenUnconnected=off
  States_hold : Outport  Port=2  OutDataTypeStr=Bus: States_Bus  VectorParamsAs1DForOutWhenUnconnected=off
  Gimbal_State_hold : Outport  Port=3  OutDataTypeStr=Bus: Gimbal_State_Bus  VectorParamsAs1DForOutWhenUnconnected=off
  External_Inputs_hold : Outport  Port=4  OutDataTypeStr=Bus: External_Inputs_Bus  VectorParamsAs1DForOutWhenUnconnected=off
  wires:
  Simulation_Control_update/1 -> Simulation_Control_hold/1
  States_update/1 -> States_hold/1
  Gimbal_State_update/1 -> Gimbal_State_hold/1
  External_Inputs_update/1 -> External_Inputs_hold/1

== system lib_GRM_HIL/FCC/Emulate_FCC/FB_Com_freq_emul ==
  update : Inport  OutDataTypeStr=Bus: FCC_Commands_Bus
  function : TriggerPort  TriggerType=function-call  VariantControl=Variant
  hold : Outport  OutDataTypeStr=Bus: FCC_Commands_Bus  VectorParamsAs1DForOutWhenUnconnected=off
  wires:
  update/1 -> hold/1

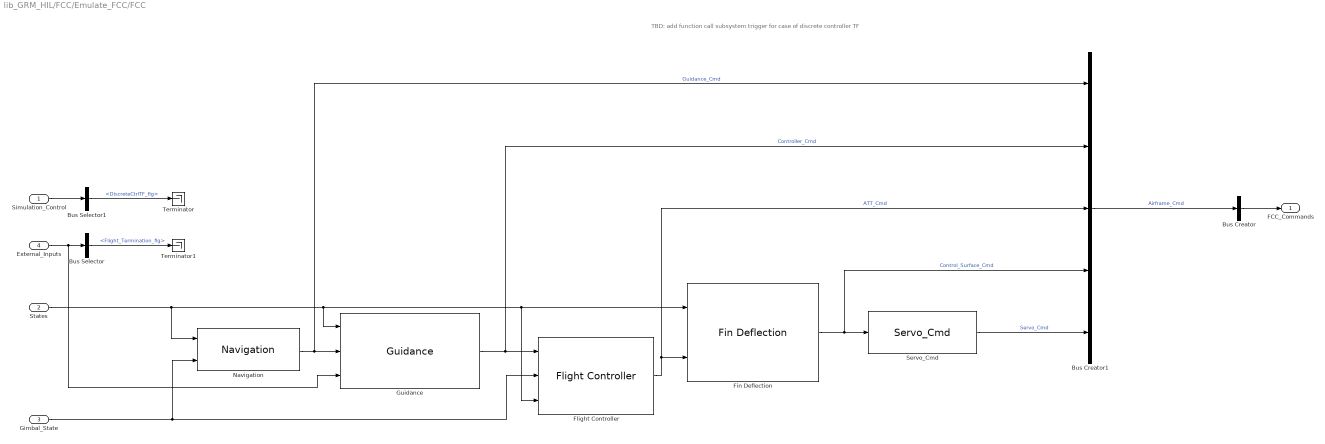
== system lib_GRM_HIL/FCC/Emulate_FCC/FCC ==
  note: TBD: add function call subsystem trigger for case of discrete controller TF
  Simulation_Control : Inport  OutDataTypeStr=Bus: Simulation_Ctrl_Bus
  States : Inport  Port=2  OutDataTypeStr=Bus: States_Bus
  Gimbal_State : Inport  Port=3  OutDataTypeStr=Bus: Gimbal_State_Bus
  External_Inputs : Inport  Port=4  OutDataTypeStr=Bus: External_Inputs_Bus
  Bus Creator : BusCreator  Inputs=1  OutDataTypeStr=Bus: FCC_Commands_Bus
  Bus Creator1 : BusCreator  Inputs=5  OutDataTypeStr=Bus: Airframe_Cmd_Bus
  Bus Selector : BusSelector  OutputSignals=FCC_External_Inputs.Flight_Termination_flg
  Bus Selector1 : BusSelector  OutputSignals=FCC_Ctrl.DiscreteCtrlTF_flg
  Fin Deflection : lib_Fin_Deflections/Fin Deflection  Control_Surfaces=HIL_Data.Control_Surfaces
  Flight Controller : lib_Flight_Controller/Flight Controller  FCC=HIL_Data.Flight_Controller
  Guidance : lib_Flight_Controller/Guidance  SystemSampleTime=-1  Latency=0  AutoFrameSizeCalculation=off
  Navigation : lib_Flight_Controller/Navigation  SystemSampleTime=-1  Latency=0  AutoFrameSizeCalculation=off
  Servo_Cmd : lib_Servo/Servo_Cmd  PWM=HIL_Data.Servo.PWM  Control_Surfaces=HIL_Data.Control_Surfaces
  Terminator : Terminator
  Terminator1 : Terminator
  FCC_Commands : Outport  OutDataTypeStr=Bus: FCC_Commands_Bus  VectorParamsAs1DForOutWhenUnconnected=off
  wires:
  Bus Selector/1 -> Terminator1/1  "<Flight_Termination_flg>"
  Flight Controller/1 -> Bus Creator1/3, Fin Deflection/2  "ATT_Cmd"
  Gimbal_State/1 -> Navigation/2, Flight Controller/2
  External_Inputs/1 -> Guidance/3, Bus Selector/1
  Bus Creator1/1 -> Bus Creator/1  "Airframe_Cmd"
  Navigation/1 -> Bus Creator1/1, Guidance/2  "Guidance_Cmd"
  States/1 -> Navigation/1, Guidance/1, Flight Controller/3, Fin Deflection/1
  Bus Creator/1 -> FCC_Commands/1
  Guidance/1 -> Bus Creator1/2, Flight Controller/1  "Controller_Cmd"
  Fin Deflection/1 -> Bus Creator1/4, Servo_Cmd/1  "Control_Surface_Cmd"
  Servo_Cmd/1 -> Bus Creator1/5  "Servo_Cmd"
  Simulation_Control/1 -> Bus Selector1/1
  Bus Selector1/1 -> Terminator/1  "<DiscreteCtrlTF_flg>"

== matlab function lib_GRM_HIL/FCC/Emulate_FCC/Com_Sync/Counter_with_external_limit ==
  data: limit input; value output; last_value input
function value = Counter(limit,last_value)
    
    if last_value < limit
        value = last_value + 1;
    else
        value = 0;
    end
    
end
